simulink model "ModelValidation"  (R2023b)
settings: Solver=VariableStepAuto  StartTime=0.0  StopTime=1  RelTol=1e-3
undefined symbols (not defined in the file): A, Adis, B, Bdis, C, Cd, Cd_book, Cdis, Cf, Cf_boook, D, Ddis, L, L1, L1_book, L_grid, L_trafo, Ld, Ld_book, R1, R1_book, R_trafo, Rd, Rd_book, Ts
libraries: spsSeriesRLCBranchLib x13, spsControlledVoltageSourceLib x4, spsThreePhaseSeriesRLCBranchLib x3, spsCurrentMeasurementLib x3, spsThreePhaseVIMeasurementLib x2, simulink x1, spsParallelRLCBranchLib x1, spsVoltageMeasurementLib x1, sps_lib x1
settings Model: Creator=uriel  LastModifiedBy=uriel
settings OptimizationCC: BlockReduction=off  ConditionallyExecuteInputs=off

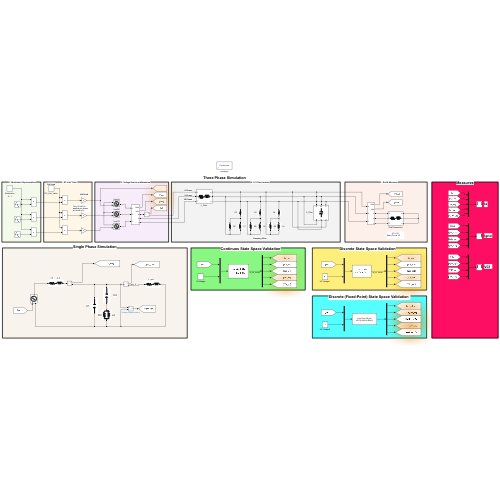
[thumbnail: Simulink's stored preview of the top-level diagram]
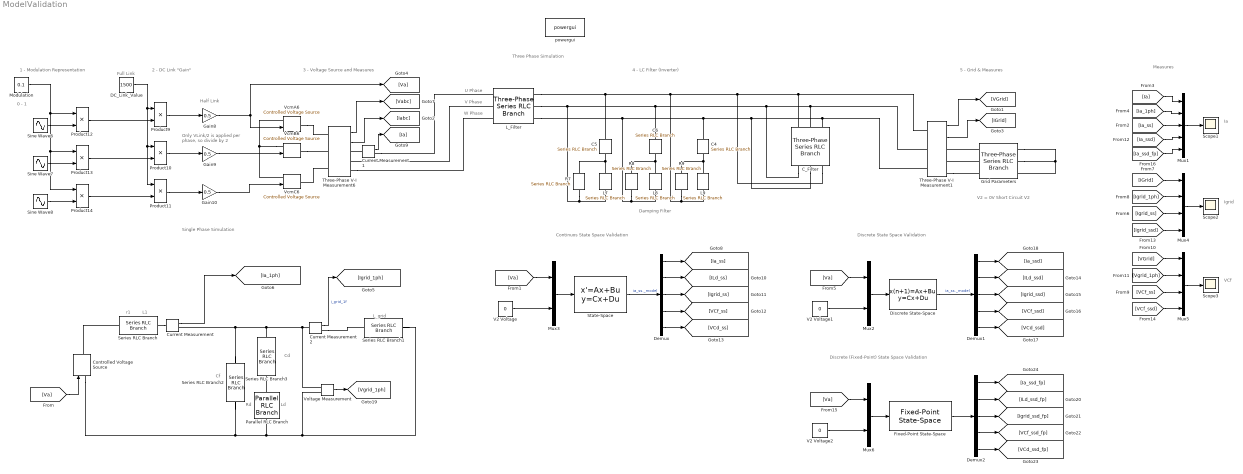
== system ModelValidation ==
  note: Ld
  note: L_grid
  note: r1
  note: Cd
  note: L1
  note: Rd
  note: Cf
  note: 1 - Modulation Representation
  note: 0 - 1
  note: 2 - DC Link "Gain"
  note: Full Link
  note: Only VLink/2 is applied per phase, so divide by 2
  note: Half Link
  note: 3 - Voltage Source and Measures
  note: U Phase
  note: V Phase
  note: W Phase
  note: Damping Filter
  note: 4 - LC Filter (Inverter)
  note: 5 - Grid & Measures
  note: V2 = 0V
      | Short Circuit V2
  note: Three Phase Simulation
  note: Continuos State Space Validation
  note: Single Phase Simulation
  note: Discrete State Space Validation
  note: Measures
  note: Ia
  note: Igrid
  note: VCf
  note: Discrete (Fixed-Point) State Space Validation
  C4 : spsSeriesRLCBranchLib/Series RLC Branch  LConnTagsString=__new0  RConnTagsString=__new0  BranchType=C  Resistance=0.001  Inductance=1e-3  SetiL0=off  InitialCurrent=0  Capacitance=Cd_book/3  Setx0=on  InitialVoltage=0  Measurements=None
  C5 : spsSeriesRLCBranchLib/Series RLC Branch  LConnTagsString=__new0  RConnTagsString=__new0  BranchType=C  Resistance=0.001  Inductance=1e-3  SetiL0=off  InitialCurrent=0  Capacitance=Cd_book/3  Setx0=on  InitialVoltage=0  Measurements=None
  C6 : spsSeriesRLCBranchLib/Series RLC Branch  LConnTagsString=__new0  RConnTagsString=__new0  BranchType=C  Resistance=0.001  Inductance=1e-3  SetiL0=off  InitialCurrent=0  Capacitance=Cd_book/3  Setx0=on  InitialVoltage=0  Measurements=None
  C_Filter : spsThreePhaseSeriesRLCBranchLib/Three-Phase Series RLC Branch  LConnTagsString=A|B|C  RConnTagsString=A|B|C  BranchType=C  Resistance=1e-3  Inductance=L  Capacitance=Cf_boook/3  Measurements=None
  Controlled Voltage Source : spsControlledVoltageSourceLib/Controlled Voltage Source  Initialize=on  Source_Type=AC  Amplitude=0  Phase=0  Frequency=0  Measurements=None
  Current Measurement : spsCurrentMeasurementLib/Current Measurement  PhasorSimulation=off  OutputType=Complex  PSBequivalent=0
  Current Measurement1 : spsCurrentMeasurementLib/Current Measurement  PhasorSimulation=off  OutputType=Complex  PSBequivalent=0
  Current Measurement2 : spsCurrentMeasurementLib/Current Measurement  PhasorSimulation=off  OutputType=Complex  PSBequivalent=0
  DC_Link_Value : Constant  Value=1500
  Demux : Demux  Outputs=5
  Demux1 : Demux  Outputs=5
  Demux2 : Demux  Outputs=5
  Discrete State-Space : DiscreteStateSpace  A=Adis  B=Bdis  C=Cdis  D=Ddis  SampleTime=Ts
  Fixed-Point State-Space : simulink/Additional Math & Discrete/Additional Discrete/Fixed-Point State-Space  A=Adis  B=Bdis  C=Cdis  D=Ddis  InitialCondition=0.0  InternalDataType=fixdt(1,32,5)  StateEqScaling=2^0  OutputEqScaling=2^0  DoSatur=off
  Gain10 : Gain  Gain=0.5
  Gain8 : Gain  Gain=0.5
  Gain9 : Gain  Gain=0.5
  Grid Parameters : spsThreePhaseSeriesRLCBranchLib/Three-Phase Series RLC Branch  LConnTagsString=A|B|C  RConnTagsString=A|B|C  BranchType=RL  Resistance=R_trafo  Inductance=L_trafo + L_grid  Capacitance=1e-6  Measurements=None
  L7 : spsSeriesRLCBranchLib/Series RLC Branch  LConnTagsString=__new0  RConnTagsString=__new0  BranchType=L  Resistance=0.001  Inductance=Ld_book*3  SetiL0=off  InitialCurrent=0  Capacitance=6000e-6  Setx0=on  InitialVoltage=156  Measurements=None
  L8 : spsSeriesRLCBranchLib/Series RLC Branch  LConnTagsString=__new0  RConnTagsString=__new0  BranchType=L  Resistance=0.001  Inductance=Ld_book*3  SetiL0=off  InitialCurrent=0  Capacitance=6000e-6  Setx0=on  InitialVoltage=156  Measurements=None
  L9 : spsSeriesRLCBranchLib/Series RLC Branch  LConnTagsString=__new0  RConnTagsString=__new0  BranchType=L  Resistance=0.001  Inductance=Ld_book*3  SetiL0=off  InitialCurrent=0  Capacitance=6000e-6  Setx0=on  InitialVoltage=156  Measurements=None
  L_Filter : spsThreePhaseSeriesRLCBranchLib/Three-Phase Series RLC Branch  LConnTagsString=A|B|C  RConnTagsString=A|B|C  BranchType=RL  Resistance=R1_book  Inductance=L1_book  Capacitance=1e-6  Measurements=None
  Modulation : Constant  Value=0.1
  Mux1 : Mux  Inputs=5
  Mux2 : Mux  Inputs=2
  Mux3 : Mux  Inputs=2
  Mux4 : Mux
  Mux5 : Mux
  Mux6 : Mux  Inputs=2
  Parallel RLC Branch : spsParallelRLCBranchLib/Parallel RLC Branch  LConnTagsString=a  RConnTagsString=__new0  BranchType=RL  Resistance=Rd  Inductance=Ld  SetiL0=off  InitialCurrent=0  Capacitance=1e-6  Setx0=off  InitialVoltage=0  Measurements=None
  Product{9..14} (6 alike) : Product
  R7 : spsSeriesRLCBranchLib/Series RLC Branch  LConnTagsString=__new0  RConnTagsString=__new0  BranchType=R  Resistance=Rd_book*3  Inductance=1e-3  SetiL0=off  InitialCurrent=0  Capacitance=6000e-6  Setx0=on  InitialVoltage=156  Measurements=None
  R8 : spsSeriesRLCBranchLib/Series RLC Branch  LConnTagsString=__new0  RConnTagsString=__new0  BranchType=R  Resistance=Rd_book*3  Inductance=1e-3  SetiL0=off  InitialCurrent=0  Capacitance=6000e-6  Setx0=on  InitialVoltage=156  Measurements=None
  R9 : spsSeriesRLCBranchLib/Series RLC Branch  LConnTagsString=__new0  RConnTagsString=__new0  BranchType=R  Resistance=Rd_book*3  Inductance=1e-3  SetiL0=off  InitialCurrent=0  Capacitance=6000e-6  Setx0=on  InitialVoltage=156  Measurements=None
  Scope1 : Scope
  Scope2 : Scope
  Scope3 : Scope
  Series RLC Branch : spsSeriesRLCBranchLib/Series RLC Branch  LConnTagsString=__new0  RConnTagsString=__new0  BranchType=RL  Resistance=R1  Inductance=L1  SetiL0=off  InitialCurrent=0  Capacitance=1e-6  Setx0=off  InitialVoltage=0  Measurements=None
  Series RLC Branch1 : spsSeriesRLCBranchLib/Series RLC Branch  LConnTagsString=__new0  RConnTagsString=__new0  BranchType=RL  Resistance=R_trafo  Inductance=L_trafo + L_grid  SetiL0=off  InitialCurrent=0  Capacitance=1e-6  Setx0=off  InitialVoltage=0  Measurements=None
  Series RLC Branch2 : spsSeriesRLCBranchLib/Series RLC Branch  LConnTagsString=__new0  RConnTagsString=__new0  BranchType=C  Resistance=1e-3  Inductance=110e-6  SetiL0=off  InitialCurrent=0  Capacitance=Cf  Setx0=off  InitialVoltage=0  Measurements=None
  Series RLC Branch3 : spsSeriesRLCBranchLib/Series RLC Branch  LConnTagsString=__new0  RConnTagsString=__new0  BranchType=C  Resistance=1e-3  Inductance=110e-6  SetiL0=off  InitialCurrent=0  Capacitance=Cd  Setx0=off  InitialVoltage=0  Measurements=None
  Sine Wave6 : Sin  Frequency=2*pi*60  SampleTime=0
  Sine Wave7 : Sin  Frequency=2*pi*60  Phase=-120*pi/180  SampleTime=0
  Sine Wave8 : Sin  Frequency=2*pi*60  Phase=120*pi/180  SampleTime=0
  State-Space : StateSpace  A=A  B=B  C=C  D=D  InitialCondition=0
  Three-Phase V-I Measurement1 : spsThreePhaseVIMeasurementLib/Three-Phase V-I Measurement  VoltageMeasurement=phase-to-phase  SetLabelV=off  LabelV=Vabc  Vpu=off  VpuLL=off  CurrentMeasurement=yes  SetLabelI=off  LabelI=Iabc  Ipu=off  Pbase=100e6  Vbase=500e3  OutputType=Complex  PhasorSimulation=off  PSBequivalent=0
  Three-Phase V-I Measurement6 : spsThreePhaseVIMeasurementLib/Three-Phase V-I Measurement  VoltageMeasurement=phase-to-phase  SetLabelV=off  LabelV=Vabc  Vpu=off  VpuLL=off  CurrentMeasurement=yes  SetLabelI=off  LabelI=Iabc  Ipu=off  Pbase=100e6  Vbase=500e3  OutputType=Complex  PhasorSimulation=off  PSBequivalent=0
  V2 Voltage : Constant  Value=0
  V2 Voltage1 : Constant  Value=0
  V2 Voltage2 : Constant  Value=0
  VcmA6 : spsControlledVoltageSourceLib/Controlled Voltage Source  Initialize=off  Source_Type=AC  Amplitude=0  Phase=0  Frequency=0  Measurements=None
  VcmB6 : spsControlledVoltageSourceLib/Controlled Voltage Source  Initialize=off  Source_Type=AC  Amplitude=0  Phase=0  Frequency=0  Measurements=None
  VcmC6 : spsControlledVoltageSourceLib/Controlled Voltage Source  Initialize=off  Source_Type=AC  Amplitude=0  Phase=0  Frequency=0  Measurements=None
  Voltage Measurement : spsVoltageMeasurementLib/Voltage Measurement  PhasorSimulation=off  OutputType=Complex  PSBequivalent=0
  powergui : sps_lib/powergui  Priority=1  SimulationMode=Continuous  SampleTime=1e-6  frequency=60  Iterations=50  frequencyindice=0  Pbase=100e6  ErrMax=1e-4  UnitsV=kV  UnitsW=MW  buscounter=0  FunctionMessages=off  echomessages=off  EnableUseOfTLC=off  CurrentSourceSwitches=off  DisableSnubberDevices=off  DisableRonSwitches=off  DisableVfSwitches=off  DisplayEquations=off  AutomaticDiscreteSolvers=off  SolverType=Tustin/Backward Euler (TBE)  Interpol=off  ExternalGateDelay=off  methode=off  Ts=100  x0status=blocks  SPID=on  SwTol=0  HookPort=off  NonlinearTolerance=1e-4  nMaxIteration=100  ContinueOnMaxIteration=off  RestoreLinks=warning  ResistiveCurrentMeasurement=off  Frange=[0:2:500]  Ylog=off  Xlog=on  ShowGrid=off  save=off  variable=ZData  structure=0  ZoomFFT=off  StartTime=0.0  cycles=1  DisplayStyle=1  fundamental=60  FreqAxis=off  MaxFrequency=1000  frequencyindicesteady=1  RmsSteady=1  display=off
  wires:
  Gain10/1 -> VcmC6/1
  Gain8/1 -> [Va], VcmA6/1
  Product12/1 -> Product9/2
  Product10/1 -> Gain9/1
  Product14/1 -> Product11/2
  Product9/1 -> Gain8/1
  Product13/1 -> Product10/2
  Three-Phase V-I Measurement6/2 -> [Iabc]
  Sine Wave8/1 -> Product14/2
  DC_Link_Value/1 -> Product11/1, Product10/1, Product9/1
  Gain9/1 -> VcmB6/1
  Sine Wave7/1 -> Product13/2
  Sine Wave6/1 -> Product12/2
  Modulation/1 -> Product14/1, Product13/1, Product12/1
  Product11/1 -> Gain10/1
  Current Measurement/1 -> [Ia_1ph]
  [Va] -> Controlled Voltage Source/1
  Three-Phase V-I Measurement1/1 -> [VGrid]
  Three-Phase V-I Measurement1/2 -> [IGrid]
  Current Measurement2/1 -> [Igrid_1ph]  "i_grid_1f"
  Mux1/1 -> Scope1/1
  [Ia] -> Mux1/1
  [Ia_1ph] -> Mux1/2
  Three-Phase V-I Measurement6/1 -> [Vabc]
  [Va] -> Mux3/1
  State-Space/1 -> Demux/1  "ia_ss._model"
  V2 Voltage/1 -> Mux3/2
  Mux3/1 -> State-Space/1
  [Ia_ss] -> Mux1/3
  Current Measurement1/1 -> [Ia]
  Demux/1 -> [Ia_ss]
  Demux/2 -> [ILd_ss]
  Demux/4 -> [VCf_ss]
  Demux/5 -> [VCd_ss]
  Demux/3 -> [Igrid_ss]
  Demux1/3 -> [Igrid_ssd]
  Demux1/2 -> [ILd_ssd]
  Demux1/5 -> [VCd_ssd]
  Demux1/1 -> [Ia_ssd]
  [Va] -> Mux2/1
  Discrete State-Space/1 -> Demux1/1  "ia_ss._model"
  V2 Voltage1/1 -> Mux2/2
  Mux2/1 -> Discrete State-Space/1
  Demux1/4 -> [VCf_ssd]
  [Igrid_ss] -> Mux4/3
  [IGrid] -> Mux4/1
  Mux4/1 -> Scope2/1
  [Igrid_1ph] -> Mux4/2
  Voltage Measurement/1 -> [Vgrid_1ph]
  [VCf_ss] -> Mux5/3
  Mux5/1 -> Scope3/1
  [Vgrid_1ph] -> Mux5/2
  [VGrid] -> Mux5/1
  [Ia_ssd] -> Mux1/4
  [Igrid_ssd] -> Mux4/4
  [VCf_ssd] -> Mux5/4
  Mux6/1 -> Fixed-Point State-Space/1
  Demux2/4 -> [VCf_ssd_fp]
  [Va] -> Mux6/1
  V2 Voltage2/1 -> Mux6/2
  Demux2/1 -> [Ia_ssd_fp]
  Demux2/2 -> [ILd_ssd_fp]
  Demux2/5 -> [VCd_ssd_fp]
  Demux2/3 -> [Igrid_ssd_fp]
  Fixed-Point State-Space/1 -> Demux2/1
  [Ia_ssd_fp] -> Mux1/5
  connections:
  VcmB6/LConn1 -- VcmC6/LConn1 -- VcmA6/LConn1
  Grid Parameters/RConn3 -- Grid Parameters/RConn1 -- Grid Parameters/RConn2
  Grid Parameters/LConn1 -- Three-Phase V-I Measurement1/RConn1
  VcmA6/RConn1 -- Three-Phase V-I Measurement6/LConn1
  Grid Parameters/LConn2 -- Three-Phase V-I Measurement1/RConn2
  Three-Phase V-I Measurement1/RConn3 -- Grid Parameters/LConn3
  VcmB6/RConn1 -- Three-Phase V-I Measurement6/LConn2
  Three-Phase V-I Measurement6/LConn3 -- VcmC6/RConn1
  Series RLC Branch2/LConn1 -- Voltage Measurement/LConn1 -- Current Measurement2/LConn1 -- Series RLC Branch3/LConn1 -- Current Measurement/RConn1
  Controlled Voltage Source/LConn1 -- Voltage Measurement/LConn2 -- Series RLC Branch1/RConn1 -- Parallel RLC Branch/RConn1 -- Series RLC Branch2/RConn1
  Current Measurement2/RConn1 -- Series RLC Branch1/LConn1
  Series RLC Branch/LConn1 -- Controlled Voltage Source/RConn1
  Parallel RLC Branch/LConn1 -- Series RLC Branch3/RConn1
  Series RLC Branch/RConn1 -- Current Measurement/LConn1
  C_Filter/LConn2 -- Three-Phase V-I Measurement1/LConn2 -- C_Filter/RConn1 -- C6/LConn1 -- L7/RConn1 -- R7/RConn1 -- L_Filter/RConn2
  R7/LConn1 -- C5/RConn1 -- L7/LConn1
  C_Filter/LConn1 -- Three-Phase V-I Measurement1/LConn1 -- C_Filter/RConn3 -- L_Filter/RConn1 -- C5/LConn1 -- R9/RConn1 -- L9/RConn1
  R9/LConn1 -- C4/RConn1 -- L9/LConn1
  R8/LConn1 -- C6/RConn1 -- L8/LConn1
  C_Filter/LConn3 -- Three-Phase V-I Measurement1/LConn3 -- C_Filter/RConn2 -- C4/LConn1 -- L_Filter/RConn3 -- L8/RConn1 -- R8/RConn1
  L_Filter/LConn2 -- Three-Phase V-I Measurement6/RConn2
  Three-Phase V-I Measurement6/RConn3 -- L_Filter/LConn3
  Current Measurement1/RConn1 -- L_Filter/LConn1
  Current Measurement1/LConn1 -- Three-Phase V-I Measurement6/RConn1
